simulink model "ClarkeParkTransformation"  (R2013a)
settings: Solver=ode45  StartTime=0.0  StopTime=10.0  RelTol=1e-3
settings Model: Creator=Jan  LastModifiedBy=Jan

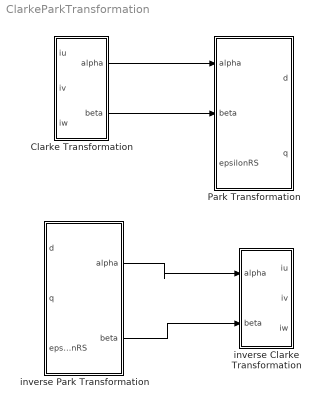
== system ClarkeParkTransformation ==
  Clarke Transformation : Subsystem
  Park Transformation : Subsystem
  inverse Clarke Transformation : Subsystem
  inverse Park Transformation : Subsystem
  wires:
  Clarke Transformation/1(alpha) -> Park Transformation/1(alpha)
  Clarke Transformation/2(beta) -> Park Transformation/2(beta)
  inverse Park Transformation/1(alpha) -> inverse Clarke Transformation/1(alpha)
  inverse Park Transformation/2(beta) -> inverse Clarke Transformation/2(beta)

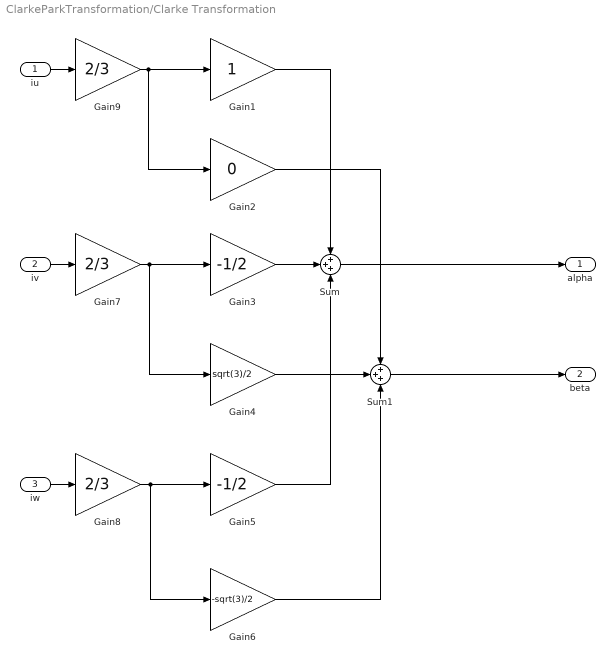
== system ClarkeParkTransformation/Clarke Transformation ==
  iu : Inport
  iv : Inport  Port=2
  iw : Inport  Port=3
  Gain1 : Gain
  "Gain2 " : Gain  Gain=0
  Gain3 : Gain  Gain=-1/2
  Gain4 : Gain  Gain=sqrt(3)/2
  Gain5 : Gain  Gain=-1/2
  Gain6 : Gain  Gain=-sqrt(3)/2
  Gain7 : Gain  Gain=2/3
  Gain8 : Gain  Gain=2/3
  Gain9 : Gain  Gain=2/3
  Sum : Sum  Inputs=+++
  Sum1 : Sum  Inputs=+++
  alpha : Outport
  beta : Outport  Port=2
  wires:
  "Gain2 "/1 -> Sum1/1
  Gain1/1 -> Sum/1
  Gain4/1 -> Sum1/2
  Gain5/1 -> Sum/3
  iw/1 -> Gain8/1
  Gain3/1 -> Sum/2
  Gain7/1 -> Gain4/1, Gain3/1
  Gain9/1 -> "Gain2 "/1, Gain1/1
  Gain8/1 -> Gain6/1, Gain5/1
  Sum/1 -> alpha/1
  Sum1/1 -> beta/1
  iv/1 -> Gain7/1
  Gain6/1 -> Sum1/3
  iu/1 -> Gain9/1

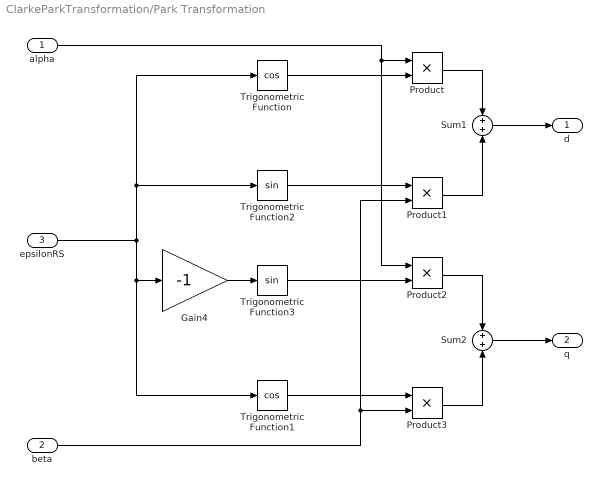
== system ClarkeParkTransformation/Park Transformation ==
  alpha : Inport
  beta : Inport  Port=2
  epsilonRS : Inport  Port=3
  Gain4 : Gain  Gain=-1
  Product{,1..3} (4 alike) : Product
  Sum1 : Sum
  Sum2 : Sum
  Trigonometric Function : Trigonometry  Operator=cos
  Trigonometric Function1 : Trigonometry  Operator=cos
  Trigonometric Function2 : Trigonometry
  Trigonometric Function3 : Trigonometry
  d : Outport
  q : Outport  Port=2
  wires:
  Sum2/1 -> q/1
  Product2/1 -> Sum2/1
  Product1/1 -> Sum1/2
  epsilonRS/1 -> Trigonometric Function2/1, Trigonometric Function/1, Gain4/1, Trigonometric Function1/1
  Trigonometric Function/1 -> Product/2
  alpha/1 -> Product2/1, Product/1
  Sum1/1 -> d/1
  Trigonometric Function1/1 -> Product3/1
  beta/1 -> Product3/2, Product1/2
  Product/1 -> Sum1/1
  Trigonometric Function2/1 -> Product1/1
  Trigonometric Function3/1 -> Product2/2
  Product3/1 -> Sum2/2
  Gain4/1 -> Trigonometric Function3/1

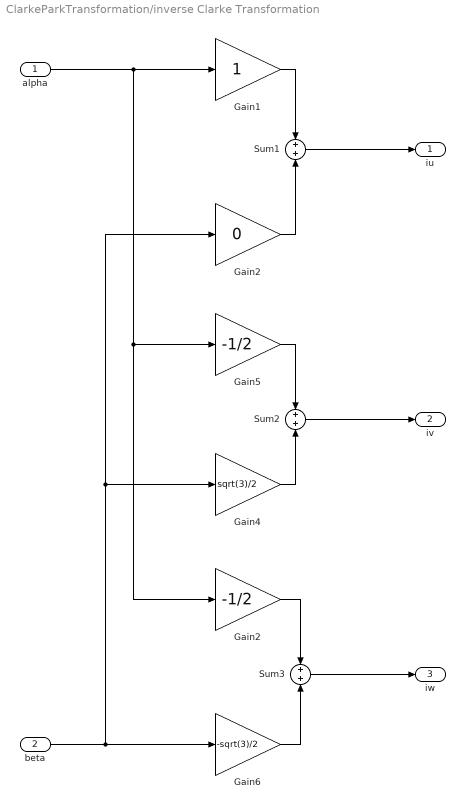
== system ClarkeParkTransformation/inverse Clarke Transformation ==
  alpha : Inport
  beta : Inport  Port=2
  Gain1 : Gain
  Gain2 : Gain  Gain=-1/2
  "Gain2 " : Gain  Gain=0
  Gain4 : Gain  Gain=sqrt(3)/2
  Gain5 : Gain  Gain=-1/2
  Gain6 : Gain  Gain=-sqrt(3)/2
  Sum1 : Sum
  Sum2 : Sum
  Sum3 : Sum
  iu : Outport
  iv : Outport  Port=2
  iw : Outport  Port=3
  wires:
  Sum2/1 -> iv/1
  beta/1 -> "Gain2 "/1, Gain4/1, Gain6/1
  Gain4/1 -> Sum2/2
  Sum1/1 -> iu/1
  "Gain2 "/1 -> Sum1/2
  Gain5/1 -> Sum2/1
  Gain1/1 -> Sum1/1
  Gain2/1 -> Sum3/1
  Gain6/1 -> Sum3/2
  alpha/1 -> Gain1/1, Gain2/1, Gain5/1
  Sum3/1 -> iw/1

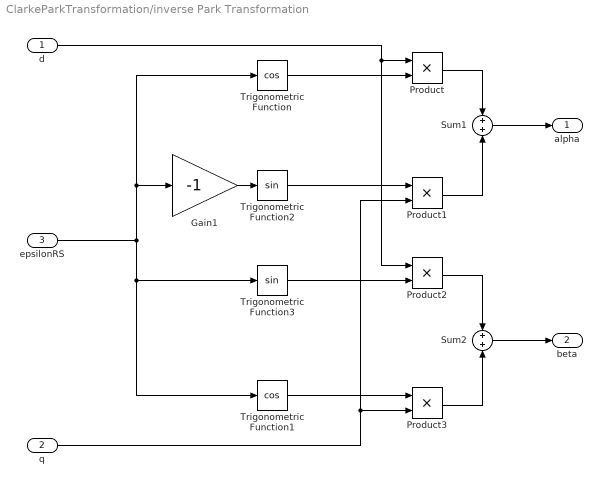
== system ClarkeParkTransformation/inverse Park Transformation ==
  d : Inport
  q : Inport  Port=2
  epsilonRS : Inport  Port=3
  Gain1 : Gain  Gain=-1
  Product{,1..3} (4 alike) : Product
  Sum1 : Sum
  Sum2 : Sum
  Trigonometric Function : Trigonometry  Operator=cos
  Trigonometric Function1 : Trigonometry  Operator=cos
  Trigonometric Function2 : Trigonometry
  Trigonometric Function3 : Trigonometry
  alpha : Outport
  beta : Outport  Port=2
  wires:
  Sum2/1 -> beta/1
  Product2/1 -> Sum2/1
  Product1/1 -> Sum1/2
  epsilonRS/1 -> Gain1/1, Trigonometric Function/1, Trigonometric Function3/1, Trigonometric Function1/1
  Trigonometric Function/1 -> Product/2
  d/1 -> Product2/1, Product/1
  Sum1/1 -> alpha/1
  Trigonometric Function1/1 -> Product3/1
  q/1 -> Product3/2, Product1/2
  Product/1 -> Sum1/1
  Trigonometric Function2/1 -> Product1/1
  Trigonometric Function3/1 -> Product2/2
  Product3/1 -> Sum2/2
  Gain1/1 -> Trigonometric Function2/1
